simulink model "VFlexP"  (R2025a)
settings: Solver=ode23tb  StartTime=0.0  StopTime=40  FixedStep=5e-5
model workspace (MAT data in the model file):
  DCop_DCBUCK : object (value not decoded)
  Grid_CCVSC_idx = [2; 3; 4; 5; 6; 7; 8; 9; 10; 11; 12]
  Grid_CCVSCs = 1
  Grid_CCVSCs_buses = 1
  Grid_CCVSCs_toM = [0 1 0 0 0 0 0 0 0 0 0 0 ... (781 elements, 71x11)]
  Grid_C_Lines = [0.1 0.1 0.1 0.1]
  Grid_Cbuses = [0.05000002 0.10000002 0.10000002 0.10000002 0.05000002]
  Grid_DC : object (value not decoded)
  Grid_DCop_DCBUCK : object (value not decoded)
  Grid_DCop_DC_PES : object (value not decoded)
  Grid_DFIGs = 1
  Grid_DFIGs_buses = 1
  Grid_DGs : string (value not decoded)
  Grid_From_buses = [1 2 4 4]
  Grid_GFls = 1
  Grid_GFls_buses = 1
  Grid_GFr_idx = [1; 2; 3]
  Grid_GFrs = 1
  Grid_GFrs_buses = 1
  Grid_GFrs_toM = [1 0 0 0 0 0 0 0 0 1 0 0 ... (15 elements, 5x3)]
  Grid_IG_idx = 1
  Grid_IGs = 1
  Grid_IGs_buses = 1
  Grid_IGs_toM = [1; 0]
  Grid_L_Lines = [0.5 0.5 0.5 0.5]
  Grid_L_Loads = [0.000959999944704 0.000156249997559 0.00154855477548]
  Grid_Lines_fromM : object (value not decoded)
  Grid_Lines_toM : object (value not decoded)
  Grid_Load_buses = [2; 3; 4]
  Grid_Load_busesDC = []
  Grid_MGES_idx = [1; 2; 3]
  Grid_MGESs = 1
  Grid_MGESs_buses = [1; 5; 3]
  Grid_MGESs_toM = [1 0 0 0 0 0 0 0 0 1 0 0 ... (15 elements, 5x3)]
  Grid_MSGs = 1
  Grid_MSGs_buses = 1
  Grid_Nbuses = 5
  Grid_PQ_gen = [3; 2; 2]
  Grid_Ploads = [1250 4000 1250]
  Grid_PloadsDC = []
  Grid_Ps_lf = [0.274439537683 0.78 0.3]
  Grid_Qloads = [0.3 0.5 0.5]
  Grid_Qs_lf = [-0.0366071562958 0.126505596722 -0.0162964024532]
  Grid_R_Lines = [0.01 0.01 0.01 0.01]
  Grid_R_Loads = [3.9999997696 1.24999998047 3.8713869387]
  Grid_R_Loads_DC = 0
  Grid_Rcf = [50000000 50000000 50000000 50000000 50000000]
  Grid_SCs = 1
  Grid_SCs_buses = 1
  Grid_SG_idx = 1
  Grid_SGs = 1
  Grid_SGs_buses = 1
  Grid_SGs_toM = [1; 0]
  Grid_To_buses = [2 3 3 5]
  Grid_VCVSC_idx = [1; 2; 3; 4; 5; 6; 7; 8; 9; 10; 11; 12]
  Grid_VCVSCs = 1
  Grid_VCVSCs_buses = [1; 2; 3; 6; 8; 9; 12; 58; 59; 60; 63; 65]
  Grid_VCVSCs_toM = [1 0 0 0 0 0 0 0 0 0 0 0 ... (852 elements, 71x12)]
  Grid_VSM_idx = [1; 2; 3]
  Grid_VSMs = 1
  Grid_VSMs_buses = 1
  Grid_VSMs_toM = [1 0 0 0 0 0 0 0 0 1 0 0 ... (15 elements, 5x3)]
  Grid_admitt_matrix = [2.15353135314-19.7953135314i  -1.9801980198+19.801980198i; -1.9801980198+19.801980198i  2.15353135314-19.7953135314i]
  Grid_admitt_matrix_noloads = [1.98686468647-19.7953135314i  -1.9801980198+19.801980198i; -1.9801980198+19.801980198i  1.98686468647-19.7953135314i]
  Grid_bus = [1; 2; 6; 7; 8]
  Grid_busDC_complexity = [1 1 1]
  Grid_busDC_complexity_PF = [2 2 2]
  Grid_bus_complexity = [1 1 1 1 1]
  Grid_bus_complexity_PF = [1 1 1 1 1]
  Grid_buses_lf = [1; 5; 3]
  Grid_conductance_matrix = [100.00000002  -100  0; -100  200.00000002  -100; 0  -100  100.00000002]
  Grid_conductance_matrix_noloads = [100.00000002  -100  0; -100  200.00000002  -100; 0  -100  100.00000002]
  Grid_fref : object (value not decoded)
  Grid_gen_static_params : mBase (value not decoded)
  Grid_iPs_lf = [3.64378984326 1.28205128205 3.33333333333]
  Grid_iQs_lf = [-27.3170631425 7.90478860943 -61.3632366329]
  Grid_iadmitt_matrix = [2.88165849328-0.0982918688642i  2.87905051706-0.123273862303i; 2.87905051706-0.123273862303i  2.88165849328-0.0982918688642i]
  Grid_iadmitt_matrix_noloads = [37.5012524798-37.4874983544i  37.4987475202-37.5125016456i; 37.4987475202-37.5125016456i  37.5012524798-37.4874983544i]
  Grid_iconductance_matrix = [16666671.4556  16666671.4489  16666671.4456; 16666671.4489  16666671.4522  16666671.4489; 16666671.4456  16666671.4489  16666671.4556]
  Grid_iconductance_matrix_noloads = [16666671.4556  16666671.4489  16666671.4456; 16666671.4489  16666671.4522  16666671.4489; 16666671.4456  16666671.4489  16666671.4556]
  Grid_init_OK_bool = 1
  Grid_intconv_PF : object (value not decoded)
  Grid_lf_op : op_report (value not decoded)
  Grid_lineDC_complexity = [1 1]
  Grid_lineDC_complexity_PF = [2 2]
  Grid_line_complexity = [1 1 1 1]
  Grid_line_complexity_PF = [3 3 3 3]
  Grid_loadDC_complexity = []
  Grid_loadDC_complexity_PF = []
  Grid_load_complexity = [3 3 3]
  Grid_load_complexity_PF = [4 4 4]
  Grid_opDC_CCVSC : object (value not decoded)
  Grid_opDC_VSM : object (value not decoded)
  Grid_opGFr : object (value not decoded)
  Grid_opVCVSC : object (value not decoded)
  Grid_op_CCVSC : object (value not decoded)
  Grid_op_IG : object (value not decoded)
  Grid_op_MGES : object (value not decoded)
  Grid_op_SG : object (value not decoded)
  Grid_op_VSM : object (value not decoded)
  Grid_shift_lines = [0 0 0 0]
  Grid_tap_lines = [1 1 1 1]
  Grid_v_buses_mod = [1 1 1 0.9837920967 1]
  LinsysParamChangeStruct : Param1 (value not decoded)
  Lline = 0.01
  Rline = 1e-05
  linsys : object (value not decoded)
symbols that are objects in the model workspace (value not decoded): Grid_DCop_DC_PES, Grid_DCop_DCBUCK, Grid_op_CCVSC, Grid_op_IG, Grid_op_MGES, Grid_op_SG, Grid_op_VSM, Grid_opDC_CCVSC, Grid_opDC_VSM, Grid_opGFr, Grid_opVCVSC
undefined symbols (not defined in the file): block_buses_DC, block_idx, CCVSC_idx, Cf, costs, costs2, D, DFIGs_nodes, DiscIntNeverNeededParam, entity, Fb, Fi, From_nodes, grid_linsys, Grid_op_DFIG, Grid_op_DFIG_PQ, Grid_op_MSG, Grid_op_SC, Grid_op_VCVSC, H, initial_states_grid, K_1, K_3, K_5, K_A, K_C, K_IM, K_IR, K_P, K_PM, K_PR, K_S1, K_S2, K_S3, Ki_w, Kic, Kiv, Kp_id, Kp_theta, Kp_w, Kpc, Kpv, last_send, Lc, Lf, Lfd, Lkd1, Lkd2, Lkq1, Lkq2, Lkq3, Lmd, Lmq, Lsd, Lsq, m, M, Matrix_flux_to_i, mp, MSGs_buses ... (+44)
libraries: simulink x1048, eeGeneralControl x12
(part 18 of 50)

== system VFlexP/Grid/Secondary Control/Matrices with delay and limitation/limitation ==
  In1 : Inport
  AND{,1..3} (4 alike) : Logic  IconShape=distinctive  AllPortsSameDT=off  OutDataTypeStr=boolean
  Assignment1 : Assignment  NumberOfDimensions=2  DiagnosticForDimensions=Warning  IndexOptions=Index vector (dialog),Assign all  Indices=2,1  OutputSizes=1,1
  Assignment2 : Assignment  NumberOfDimensions=2  DiagnosticForDimensions=Warning  IndexOptions=Index vector (dialog),Assign all  Indices=4,1  OutputSizes=1,1
  Assignment3 : Assignment  DiagnosticForDimensions=Warning  IndexOptions=Index vector (port)  Indices=4  OutputSizes=1
  Assignment4 : Assignment  DiagnosticForDimensions=Warning  IndexOptions=Index vector (port)  Indices=4  OutputSizes=1
  Cast To Double : DataTypeConversion  OutDataTypeStr=double  SaturateOnIntegerOverflow=off  RndMeth=Floor
  Cast To Double1 : DataTypeConversion  OutDataTypeStr=double  SaturateOnIntegerOverflow=off  RndMeth=Floor
  Compare To Zero : simulink/Logic and Bit Operations/Compare To Zero  relop=>  OutDataTypeStr=boolean
  Compare To Zero1 : simulink/Logic and Bit Operations/Compare To Zero  relop=<  OutDataTypeStr=boolean
  Compare To Zero2 : simulink/Logic and Bit Operations/Compare To Zero  relop=>  OutDataTypeStr=boolean
  Compare To Zero3 : simulink/Logic and Bit Operations/Compare To Zero  relop=<  OutDataTypeStr=boolean
  Constant1 : Constant  Value=max(Qs_lf)*20  VectorParams1D=off
  Constant2 : Constant  Value=0.02  VectorParams1D=off
  Constant3 : Constant  Value=0.02  VectorParams1D=off
  Gain1 : Gain  Gain=-1
  Matrix Concatenate1 : Concatenate  NumInputs=4  Mode=Multidimensional array
  NOT : Logic  Operator=NOT  IconShape=distinctive  AllPortsSameDT=off  OutDataTypeStr=boolean
  NOT1 : Logic  Operator=NOT  IconShape=distinctive  AllPortsSameDT=off  OutDataTypeStr=boolean
  OR : Logic  Operator=OR  IconShape=distinctive  AllPortsSameDT=off  OutDataTypeStr=boolean
  OR1 : Logic  Operator=OR  IconShape=distinctive  AllPortsSameDT=off  OutDataTypeStr=boolean
  One2 : Constant  Value=zeros(1, length(buses_lf))  VectorParams1D=off  OutDataTypeStr=Inherit: Inherit via back propagation
  One3 : Constant  Value=ones(1, length(buses_lf))  VectorParams1D=off  OutDataTypeStr=Inherit: Inherit via back propagation
  One4 : Constant  OutDataTypeStr=Inherit: Inherit via back propagation
  Relational Operator : RelationalOperator  Operator=>  OutDataTypeStr=boolean  RndMeth=Simplest  InputSameDT=off
  Relational Operator1 : RelationalOperator  Operator=<  OutDataTypeStr=boolean  RndMeth=Simplest  InputSameDT=off
  Relational Operator2 : RelationalOperator  Operator=>  OutDataTypeStr=boolean  RndMeth=Simplest  InputSameDT=off
  Relational Operator3 : RelationalOperator  Operator=<  OutDataTypeStr=boolean  RndMeth=Simplest  InputSameDT=off
  Saturation Dynamic : simulink/Discontinuities/Saturation Dynamic  OutMin=[]  OutMax=[]  OutDataTypeStr=Inherit: Same as second input  OutDataType=fixdt(1, 16)  OutScaling=2^-10  DoSatur=off
  Saturation Dynamic1 : simulink/Discontinuities/Saturation Dynamic  OutMin=[]  OutMax=[]  OutDataTypeStr=Inherit: Same as second input  OutDataType=fixdt(1, 16)  OutScaling=2^-10  DoSatur=off
  Selector1 : Selector  NumberOfDimensions=2  InputPortWidth=3  IndexOptions=Index vector (dialog),Select all  Indices=4,1  OutputSizes=1,1
  Selector12 : Selector  NumberOfDimensions=2  InputPortWidth=3  IndexOptions=Index vector (dialog),Select all  Indices=2,1  OutputSizes=1,1
  Sum1 : Sum  Inputs=|+-
  Sum2 : Sum  Inputs=|--
  Sum8 : Sum  Inputs=|+-
  Switch : Switch  Criteria=u2 > Threshold  SaturateOnIntegerOverflow=off  InputSameDT=off
  Zero : Constant  Value=0  OutDataTypeStr=Inherit: Inherit via back propagation
  Out1 : Outport
  Out2 : Outport  Port=2
  wires:
  Relational Operator1/1 -> AND1/1
  Compare To Zero/1 -> AND/2
  Compare To Zero1/1 -> AND1/2
  Selector12/1 -> Relational Operator1/1, Relational Operator/1, Saturation Dynamic/2, Compare To Zero1/1, Compare To Zero/1
  Sum8/1 -> Saturation Dynamic/1
  [Pref] -> Sum8/2
  AND1/1 -> OR/2
  AND/1 -> OR/1
  OR/1 -> NOT/1
  Sum2/1 -> Saturation Dynamic/3
  Relational Operator/1 -> AND/1
  Saturation Dynamic/1 -> Assignment1/2, Relational Operator1/2, Relational Operator/2
  Constant2/1 -> Sum8/1
  NOT/1 -> Cast To Double/1
  Cast To Double/1 -> Matrix Concatenate1/2
  Assignment1/1 -> Assignment2/1
  Saturation Dynamic1/1 -> Assignment2/2, Relational Operator3/2, Relational Operator2/2
  Constant1/1 -> Sum1/1
  NOT1/1 -> Cast To Double1/1
  [Qref] -> Sum1/2
  Relational Operator2/1 -> AND2/1
  AND3/1 -> OR1/2
  Gain1/1 -> Saturation Dynamic1/3
  OR1/1 -> NOT1/1
  Selector1/1 -> Relational Operator3/1, Relational Operator2/1, Saturation Dynamic1/2, Compare To Zero3/1, Compare To Zero2/1
  Relational Operator3/1 -> AND3/1
  AND2/1 -> OR1/1
  Sum1/1 -> Saturation Dynamic1/1
  Compare To Zero3/1 -> AND3/2
  [Qref] -> Gain1/1
  In1/1 -> Selector1/1, Selector12/1, Assignment1/1
  Cast To Double1/1 -> Assignment4/1
  Compare To Zero2/1 -> AND2/2
  Matrix Concatenate1/1 -> Out1/1, Switch/2
  Assignment2/1 -> Switch/3, Switch/1
  Switch/1 -> Out2/1
  One3/1 -> Matrix Concatenate1/1
  Assignment3/1 -> Matrix Concatenate1/3
  [leader] -> Assignment4/3, Assignment3/3
  One2/1 -> Assignment3/1
  One4/1 -> Assignment3/2
  Assignment4/1 -> Matrix Concatenate1/4
  Zero/1 -> Assignment4/2
  [Pref] -> Sum2/1
  Constant3/1 -> Sum2/2

== system VFlexP/Grid/Secondary Control/Matrices1/Triggered Subsystem ==
  In1 : Inport
  Trigger : TriggerPort  VariantControl=(inherit)
  One : Constant  OutDataTypeStr=Inherit: Inherit via back propagation
  Sum : Sum  Inputs=|++
  Out1 : Outport
  wires:
  In1/1 -> Sum/1
  One/1 -> Sum/2
  Sum/1 -> Out1/1

== system VFlexP/Grid/Secondary Control/Matrices1/saturation_P ==
  Pref : Inport
  in : Inport  Port=2
  gaincost : Inport  Port=3
  A_P_SC : Inport  Port=4
  Constant2 : Constant  Value=0.8
  Gain12 : Gain  Gain=-1
  Product1 : Product
  Product2 : Product
  Product3 : Product
  Saturation Dynamic : simulink/Discontinuities/Saturation Dynamic  OutMin=[]  OutMax=[]  OutDataTypeStr=Inherit: Same as second input  OutDataType=fixdt(1, 16)  OutScaling=2^-10  DoSatur=off
  Sum of Elements : Sum  Inputs=+  CollapseMode=Specified dimension  CollapseDim=2
  Sum8 : Sum  Inputs=|+-
  Transpose : Math  Operator=transpose
  out : Outport
  wires:
  Pref/1 -> Sum8/2, Gain12/1
  Product1/1 -> Saturation Dynamic/1
  Product2/1 -> Saturation Dynamic/3
  Constant2/1 -> Sum8/1
  in/1 -> Saturation Dynamic/2
  Product3/1 -> Product2/2, Product1/2
  Saturation Dynamic/1 -> out/1  "out"
  Sum8/1 -> Product1/1
  Gain12/1 -> Product2/1
  A_P_SC/1 -> Sum of Elements/1
  gaincost/1 -> Product3/2
  Sum of Elements/1 -> Transpose/1
  Transpose/1 -> Product3/1

== system VFlexP/Grid/Secondary Control/Matrices1/saturation_P2 ==
  Pref : Inport
  in : Inport  Port=2
  Constant2 : Constant  Value=0.8
  Gain12 : Gain  Gain=-1
  Saturation Dynamic : simulink/Discontinuities/Saturation Dynamic  OutMin=[]  OutMax=[]  OutDataTypeStr=Inherit: Same as second input  OutDataType=fixdt(1, 16)  OutScaling=2^-10  DoSatur=off
  Sum8 : Sum  Inputs=|+-
  out : Outport
  wires:
  Pref/1 -> Sum8/2, Gain12/1
  Sum8/1 -> Saturation Dynamic/1
  Gain12/1 -> Saturation Dynamic/3
  Constant2/1 -> Sum8/1
  in/1 -> Saturation Dynamic/2
  Saturation Dynamic/1 -> out/1  "out"

== system VFlexP/Grid/Secondary Control/Pilot nodes/PI ==
  Input : Inport
  Gain : Gain
  Gain1 : Gain  Gain=10
  I : Integrator
  Sum10 : Sum  Inputs=|++
  Out1 : Outport
  wires:
  Input/1 -> Gain1/1, Gain/1
  Sum10/1 -> Out1/1
  Gain/1 -> Sum10/1
  I/1 -> Sum10/2
  Gain1/1 -> I/1

== system VFlexP/Grid/Secondary Control/Pilot nodes/PI1 ==
  Input : Inport
  Gain : Gain
  Gain1 : Gain  Gain=10
  I : Integrator
  Sum10 : Sum  Inputs=|++
  Out1 : Outport
  wires:
  Gain1/1 -> I/1
  I/1 -> Sum10/2
  Gain/1 -> Sum10/1
  Sum10/1 -> Out1/1
  Input/1 -> Gain/1, Gain1/1

== system VFlexP/Grid/Secondary Control/Pilot nodes/PLL ==
  out_q : Inport
  Gain : Gain
  Gain1 : Gain  Gain=20
  I : Integrator  InitialCondition=1
  Sum10 : Sum  Inputs=|++
  Input2 : Outport
  wires:
  I/1 -> Sum10/2
  Gain/1 -> Sum10/1
  Gain1/1 -> I/1
  out_q/1 -> Gain/1, Gain1/1
  Sum10/1 -> Input2/1

== system VFlexP/Grid/Secondary Control/Pilot nodes/Reference frame transform3 ==
  in_d : Inport
  theta : Inport  Port=2
  in_q : Inport  Port=3
  Complex to Real-Imag : ComplexToRealImag
  Cos : Trigonometry  SCDEnableBlockLinearizationSpecification=on  Operator=cos
  Product : Product
  Real-Imag to Complex : RealImagToComplex
  Real-Imag to Complex1 : RealImagToComplex
  Sin : Trigonometry  SCDEnableBlockLinearizationSpecification=on
  out_d : Outport
  out_q : Outport  Port=2
  wires:
  Complex to Real-Imag/2 -> out_q/1
  Real-Imag to Complex1/1 -> Product/1
  Real-Imag to Complex/1 -> Product/2
  Product/1 -> Complex to Real-Imag/1
  theta/1 -> Sin/1, Cos/1
  Cos/1 -> Real-Imag to Complex1/1
  Sin/1 -> Real-Imag to Complex1/2
  Complex to Real-Imag/1 -> out_d/1
  in_q/1 -> Real-Imag to Complex/2
  in_d/1 -> Real-Imag to Complex/1

== system VFlexP/Grid/Tertiary Control/MAS edp/Subsystem ==
  costs : Inport
  costs2 : Inport  Port=2
  Pmax : Inport  Port=3
  Pmin : Inport  Port=4
  x0 : Inport  Port=5
  start : Inport  Port=6
  Clock : Clock
  Compare To Constant : simulink/Logic and Bit Operations/Compare To Constant  relop=>  const=30  OutDataTypeStr=boolean
  Delay : Memory
  Delay1 : Memory
  Delay2 : Memory
  Gain : Gain  Gain=A  Multiplication=Matrix(K*u)
  Gain1 : Gain  Gain=gainM
  Gain2 : Gain  Gain=sum(A, 2)
  Gain3 : Gain  Gain=1./sum(A, 2)
  Gain4 : Gain  Gain=1/gainM
  Gain5 : Gain  Gain=-1
  Gain6 : Gain  Gain=1./sum(A, 2)
  Gain7 : Gain  Gain=2
  Memory{,1..3,5,7} (6 alike) : Memory
  NOT : Logic  Operator=NOT  IconShape=distinctive  AllPortsSameDT=off  OutDataTypeStr=boolean
  One : Constant  OutDataTypeStr=Inherit: Inherit via back propagation
  Product{,1..3} (4 alike) : Product
  Pulse Generator1 : DiscretePulseGenerator  PulseType=Time based  Period=0.1  PulseWidth=50
  Saturation Dynamic : simulink/Discontinuities/Saturation Dynamic  OutMin=[]  OutMax=[]  OutDataTypeStr=Inherit: Same as second input  OutDataType=fixdt(1, 16)  OutScaling=2^-10  DoSatur=off
  Scope{,1..3,5..6} (6 alike) : Scope
      Scope settings: ActiveDisplayYMinimum=-0.00375  ActiveDisplayYMaximum=0.03375
      Scope1 settings: ActiveDisplayYMinimum=-0.00119  ActiveDisplayYMaximum=0.00113
      Scope2 settings: ActiveDisplayYMinimum=-0.00492  ActiveDisplayYMaximum=0.03442  DataLoggingVariableName=ScopeData2
      Scope3 settings: ActiveDisplayYMinimum=-0.01846  ActiveDisplayYMaximum=0.16617  DataLoggingVariableName=ScopeData3
      Scope5 settings: ActiveDisplayYMinimum=-0.01822  ActiveDisplayYMaximum=0.06371
      Scope6 settings: ActiveDisplayYMinimum=-0.00114  ActiveDisplayYMaximum=0.00091  DataLoggingVariableName=ScopeData2
  Scope4 : Scope  NumInputPorts=2
      settings: ActiveDisplayYMinimum=-1  ActiveDisplayYMaximum=1  DataLoggingVariableName=ScopeData4
  Subsystem : Subsystem
  Sum : Sum  Inputs=|+-
  Sum of Elements : Sum  Inputs=+
  Sum of Elements1 : Sum  Inputs=+
  Sum{1..4,6,10} (6 alike) : Sum  Inputs=|++
  Sum5 : Sum  Inputs=|-+
  Sum8 : Sum  Inputs=|+-
  Sum9 : Sum  Inputs=|-+
  Switch1 : Switch  Criteria=u2 > Threshold  SaturateOnIntegerOverflow=off  InputSameDT=off
  Switch2 : Switch  Criteria=u2 ~= 0  SaturateOnIntegerOverflow=off  InputSameDT=off
  Triggered Subsystem : Subsystem  TreatAsAtomicUnit=on
  Triggered Subsystem1 : Subsystem  TreatAsAtomicUnit=on
  Triggered Subsystem2 : Subsystem  TreatAsAtomicUnit=on
  Triggered Subsystem3 : Subsystem  TreatAsAtomicUnit=on
  Triggered Subsystem4 : Subsystem  TreatAsAtomicUnit=on
  Triggered Subsystem5 : Subsystem  TreatAsAtomicUnit=on
  Triggered Subsystem6 : Subsystem  TreatAsAtomicUnit=on
  Triggered Subsystem7 : Subsystem  TreatAsAtomicUnit=on
  Zero-Order Hold : ZeroOrderHold  SampleTime=0.1
  Zero-Order Hold1 : ZeroOrderHold  SampleTime=0.1
  Pref : Outport
  wires:
  Gain/1 -> Gain3/1, Sum/1
  Switch1/1 -> Delay/1
  [sat_wup] -> Delay1/1
  [Pmin] -> Saturation Dynamic/3
  Saturation Dynamic/1 -> Sum5/1, Subsystem/2(In2), Scope/1, [P]
  Zero-Order Hold1/1 -> Memory5/1
  [P] -> Zero-Order Hold1/1
  [sat_wup] -> Memory7/1
  Gain3/1 -> Switch1/1
  Gain2/1 -> Sum/2
  Delay2/1 -> Sum3/2
  Delay1/1 -> Switch1/2
  Zero-Order Hold/1 -> Memory2/1
  Subsystem/1(Out1) -> [sat_wup]
  Gain6/1 -> Delay2/1
  Memory7/1 -> NOT/1
  [Pmax] -> Saturation Dynamic/1
  Gain4/1 -> Gain6/1
  Product1/1 -> Gain7/1
  [extra_satur] -> Gain4/1
  Product3/1 -> Triggered Subsystem1/1(In1)
  Sum3/1 -> Gain/1
  Gain7/1 -> Sum4/2
  Sum/1 -> Gain1/1
  NOT/1 -> Product3/2
  Memory1/1 -> Sum10/2, Switch2/3
  Sum10/1 -> Saturation Dynamic/2, Sum5/2, Subsystem/1(In1)
  Product/1 -> Triggered Subsystem1/Trigger
  Pmax/1 -> [Pmax]
  Pmin/1 -> [Pmin]
  [Pmin] -> Subsystem/4(Pmin)
  [Pmax] -> Subsystem/5(Pmax)
  Sum2/1 -> Product1/2
  Memory5/1 -> Sum2/1
  [x0] -> Sum2/2
  Delay/1 -> Sum3/1
  Triggered Subsystem/1(Out1) -> Scope5/1, Sum1/2
  [x0] -> Sum8/1
  Sum8/1 -> Triggered Subsystem/1(In1)
  Memory/1 -> Sum8/2
  start/1 -> [start]
  [start] -> Triggered Subsystem/Trigger
  Sum1/1 -> Scope2/1, Sum10/1
  [start] -> Triggered Subsystem2/Trigger
  Clock/1 -> Sum9/2, Triggered Subsystem2/1(In1)
  Triggered Subsystem2/1(Out1) -> Sum9/1
  Sum9/1 -> Compare To Constant/1
  Compare To Constant/1 -> Triggered Subsystem3/Trigger
  Triggered Subsystem3/1(Output) -> Pref/1
  [P] -> Triggered Subsystem3/1(In1)
  Triggered Subsystem1/1(Out1) -> Memory/1, Sum1/1
  Triggered Subsystem4/1(Out1) -> Product/2
  One/1 -> Triggered Subsystem4/1(In1)
  [start] -> Triggered Subsystem4/Trigger
  Pulse Generator1/1 -> Product/1
  Sum4/1 -> Switch1/3, Gain2/1
  Memory2/1 -> Scope1/1
  Switch2/1 -> Memory1/1
  Gain5/1 -> Switch2/2, Switch2/1
  Product2/1 -> Zero-Order Hold/1, Gain5/1
  [start] -> Triggered Subsystem7/Trigger, Triggered Subsystem6/Trigger, Triggered Subsystem5/Trigger
  x0/1 -> Triggered Subsystem5/1(x0)
  Triggered Subsystem5/1(Out1) -> [x0]
  Sum5/1 -> Product2/1
  [start] -> Memory3/1
  Memory3/1 -> Product2/2
  Sum of Elements/1 -> Scope4/1, Sum6/1
  [x0] -> Sum of Elements1/1
  [P] -> Sum of Elements/1
  Sum of Elements1/1 -> Scope4/2, Sum6/2
  Sum6/1 -> Scope3/1
  Gain1/1 -> Product3/1, Scope6/1, Subsystem/3(u)
  costs/1 -> Triggered Subsystem6/1(in)
  Triggered Subsystem6/1(out) -> Sum4/1
  costs2/1 -> Triggered Subsystem7/1(in)
  Triggered Subsystem7/1(out) -> Product1/1
